simulink model "performCoSimulationWithGazebo"  (R2023a)
settings: Solver=VariableStepAuto  StartTime=0.0  StopTime=1  RelTol=1e-3
undefined symbols (not defined in the file or in its folder): duration, force_type, fz, link, link_name, model_name, torque_type, unit_box
libraries: robotgazebolib x8
settings Model: DataDictionary=performCoSimulationWithGazeboDD.sldd  Creator=The MathWorks, Inc.  LastModifiedBy=The MathWorks, Inc.
settings SolverCC: AlgebraicLoopSolver=TrustRegion
settings DebuggingCC: UnconnectedInputMsg=warning  UnconnectedOutputMsg=warning  UnconnectedLineMsg=warning  SymbolicDimsDataTypeCodeGenerationDiagnostic=none
settings ModelReferenceCC: EnableRefExpFcnMdlSchedulingChecks=on

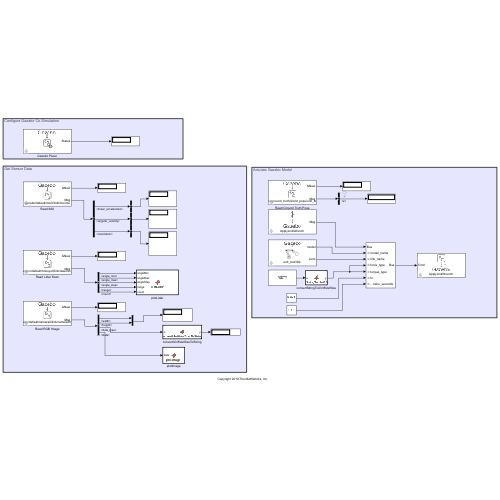
[thumbnail: Simulink's stored preview of the top-level diagram]
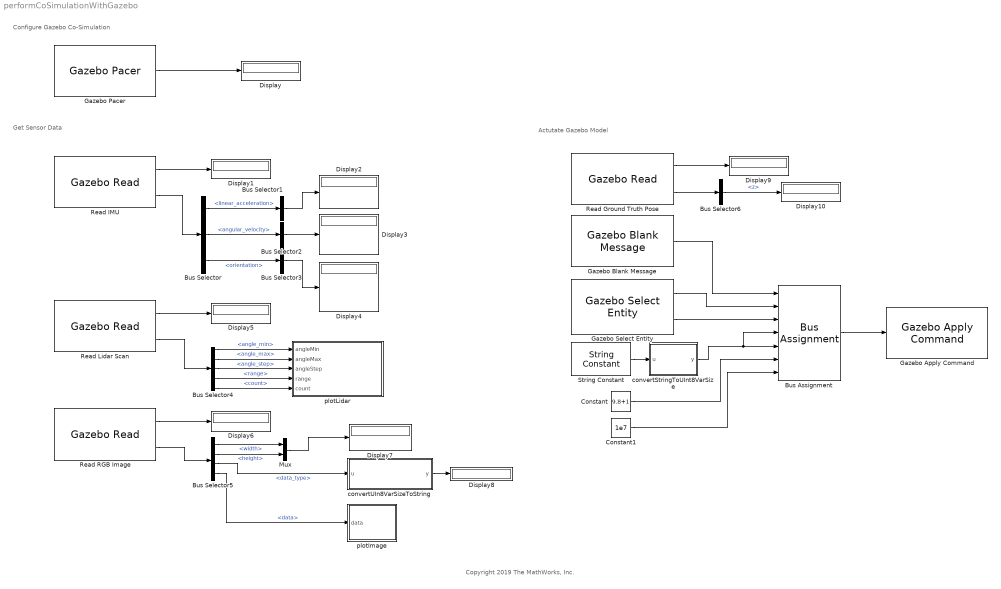
== system performCoSimulationWithGazebo ==
  note: Configure Gazebo Co-Simulation
  note: Actutate Gazebo Model
  note: Get Sensor Data
  note: Copyright 2019 The MathWorks, Inc.
  Bus Assignment : BusAssignment  AssignedSignals=model_name,link_name,force_type,torque_type,fz,duration.nano_seconds
  Bus Selector : BusSelector  OutputSignals=linear_acceleration,angular_velocity,orientation
  Bus Selector1 : BusSelector  OutputSignals=x,y,z  OutputAsBus=on
  Bus Selector2 : BusSelector  OutputSignals=x,y,z  OutputAsBus=on
  Bus Selector3 : BusSelector  OutputSignals=w,x,y,z  OutputAsBus=on
  Bus Selector4 : BusSelector  OutputSignals=angle_min,angle_max,angle_step,range,count
  Bus Selector5 : BusSelector  OutputSignals=width,height,data_type,data
  Bus Selector6 : BusSelector  OutputSignals=position.z
  Constant : Constant  Value=9.8+1
  Constant1 : Constant  Value=1e7
  Display{,1..10} (11 alike) : Display
  Gazebo Apply Command : robotgazebolib/Gazebo Apply Command  cmdType=ApplyLinkWrench  sampleTime=0.01
  Gazebo Blank Message : robotgazebolib/Gazebo Blank Message  msgType=ApplyLinkWrench  sampleTime=0.01  busName='Gazebo_SL_Bus_gazebo_msgs_ApplyLinkWrench'
  Gazebo Pacer : robotgazebolib/Gazebo Pacer  ResetBehavior=Reset Gazebo simulation time and scene  SampleTime=0.01
  Gazebo Select Entity : robotgazebolib/Gazebo Select Entity  modelElemName=unit_box/link  outputArraySize=128  OutputLabel=Joint  SelectType=Joint
  Mux : Mux  Inputs=2
  Read Ground Truth Pose : robotgazebolib/Gazebo Read  topicSource=From Gazebo  topic=/gazebo/ground_truth/world_pose/unit_box/link  messageType=gazebo_msgs/Pose  sampleTime=0.01  fixedAxisBusStatus=off  jointAxisCount=2
  Read IMU : robotgazebolib/Gazebo Read  topicSource=From Gazebo  topic=/gazebo/default/imu0/link/imu/imu  messageType=gazebo_msgs/IMU  sampleTime=0.01  fixedAxisBusStatus=off  jointAxisCount=2
  Read Lidar Scan : robotgazebolib/Gazebo Read  topicSource=From Gazebo  topic=/gazebo/default/hokuyo0/link/laser/scan  messageType=gazebo_msgs/LaserScan  sampleTime=0.01  fixedAxisBusStatus=off  jointAxisCount=2
  Read RGB Image : robotgazebolib/Gazebo Read  topicSource=From Gazebo  topic=/gazebo/default/camera0/link/camera/image  messageType=gazebo_msgs/Image  sampleTime=0.1  fixedAxisBusStatus=off  jointAxisCount=2
  String Constant : StringConstant  String="\"SET\""
  convertStringToUInt8VarSize : MATLAB Function  TreatAsAtomicUnit=on
  convertUIn8VarSizeToString : MATLAB Function  TreatAsAtomicUnit=on
  plotImage : MATLAB Function  TreatAsAtomicUnit=on
  plotLidar : MATLAB Function  TreatAsAtomicUnit=on
  wires:
  Gazebo Pacer/1 -> Display/1
  Read IMU/1 -> Display1/1
  Read IMU/2 -> Bus Selector/1
  Bus Selector/1 -> Bus Selector1/1  "<linear_acceleration>"
  Bus Selector1/1 -> Display2/1
  Bus Selector/2 -> Bus Selector2/1  "<angular_velocity>"
  Bus Selector2/1 -> Display3/1
  Bus Selector/3 -> Bus Selector3/1  "<orientation>"
  Bus Selector3/1 -> Display4/1
  Read Lidar Scan/1 -> Display5/1
  Read Lidar Scan/2 -> Bus Selector4/1
  Bus Selector4/1 -> plotLidar/1(angleMin)  "<angle_min>"
  Bus Selector4/2 -> plotLidar/2(angleMax)  "<angle_max>"
  Bus Selector4/3 -> plotLidar/3(angleStep)  "<angle_step>"
  Bus Selector4/4 -> plotLidar/4(range)  "<range>"
  Bus Selector4/5 -> plotLidar/5(count)  "<count>"
  Read RGB Image/1 -> Display6/1
  Read RGB Image/2 -> Bus Selector5/1
  Mux/1 -> Display7/1
  Bus Selector5/1 -> Mux/1  "<width>"
  Bus Selector5/2 -> Mux/2  "<height>"
  Bus Selector5/3 -> convertUIn8VarSizeToString/1(u)  "<data_type>"
  convertUIn8VarSizeToString/1(y) -> Display8/1
  Bus Selector5/4 -> plotImage/1(data)  "<data>"
  Read Ground Truth Pose/1 -> Display9/1
  Read Ground Truth Pose/2 -> Bus Selector6/1
  Bus Selector6/1 -> Display10/1  "<z>"
  Gazebo Blank Message/1 -> Bus Assignment/1
  Bus Assignment/1 -> Gazebo Apply Command/1
  Gazebo Select Entity/1 -> Bus Assignment/2
  Gazebo Select Entity/2 -> Bus Assignment/3
  String Constant/1 -> convertStringToUInt8VarSize/1(u)
  convertStringToUInt8VarSize/1(y) -> Bus Assignment/5, Bus Assignment/4
  Constant1/1 -> Bus Assignment/7
  Constant/1 -> Bus Assignment/6

== matlab function performCoSimulationWithGazebo/convertUIn8VarSizeToString ==
  data: u input; y output string
function y = convertUInt8VarSizeToString(u)

y = convertCharsToStrings(char(u'));

== matlab function performCoSimulationWithGazebo/plotLidar ==
  data: angleMin input; angleMax input; angleStep input; range input; count input
function plotLidar(angleMin, angleMax, angleStep, range, count)
%plotLidar plot Lidar Scans
coder.extrinsic('lidarScan');
coder.extrinsic('plot');

persistent h

if isempty(h)
    h = newplot(figure());
end

if count ~= 0
    plot(lidarScan(range, angleMin:angleStep:angleMax), 'Parent', h);
    grid(h, 'on');
    axis(h, 'equal');
    view(h, -90, 90);
    xlabel(h, 'X');
    ylabel(h, 'Y');
end

end

== matlab function performCoSimulationWithGazebo/plotImage ==
  data: data input
function plotImage(data)

coder.extrinsic('imshow');
coder.extrinsic('helperPlotImage');

persistent h

if isempty(h)
    h = newplot(figure());
end


y = zeros(240, 320, 3, 'uint8');
if ~isempty(data) && ~isscalar(data)
    y(:) = helperPlotImage(data);
end
imshow(y, 'Parent', h);

== matlab function performCoSimulationWithGazebo/convertStringToUInt8VarSize ==
  data: u input; y output size=128
function y = convertStringToUInt8VarSize(u)

y = uint8(convertStringsToChars(u))';
